simulink model "DiagramaDeSimulacao"  (R2019a)
settings: Solver=VariableStepAuto  StartTime=0.0  StopTime=210  RelTol=1e-3
values from neighbouring files (symbols this model uses):
  k1 = 6.01    [scriptDeSimulacao.m]
  k2 = 0.8433    [scriptDeSimulacao.m]
  k3 = 0.1123    [scriptDeSimulacao.m]
  V = 100    [scriptDeSimulacao.m]
libraries: powerlib_meascontrol x1
settings Model: Creator=Usuario  LastModifiedBy=Usuario

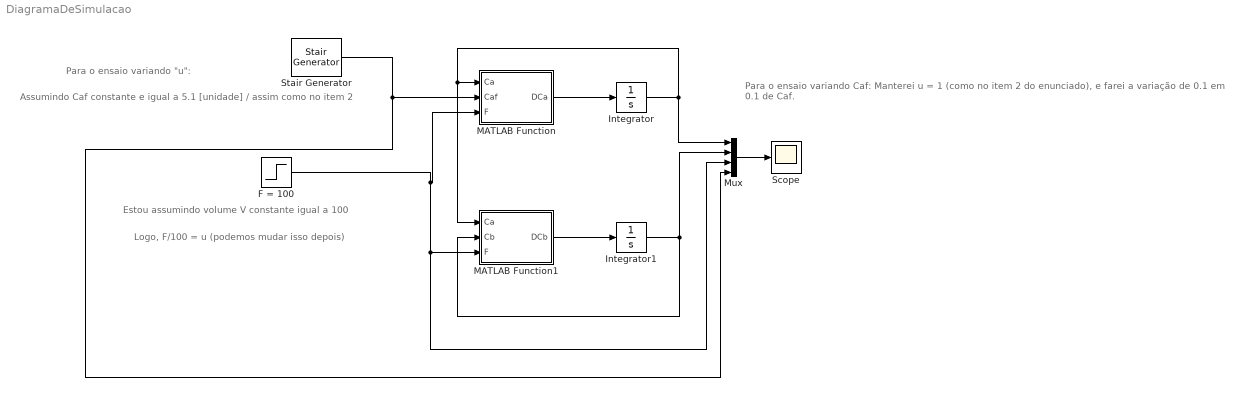
== system DiagramaDeSimulacao ==
  note: Para o ensaio variando Caf: Manterei u = 1 (como no item 2 do enunciado), e farei a variação de 0.1 em 0.1 de Caf.
  note: Para o ensaio variando "u":
  note: Assumindo Caf constante e igual a 5.1 [unidade] / assim como no item 2
  note: Logo, F/100 = u (podemos mudar isso depois)
  note: Estou assumindo volume V constante igual a 100
  F = 100 : Step  Time=0  After=100  SampleTime=0
  Integrator : Integrator
  Integrator1 : Integrator
  MATLAB Function : MATLAB Function  TreatAsAtomicUnit=on
  MATLAB Function1 : MATLAB Function  TreatAsAtomicUnit=on
  Mux : Mux
  Scope : Scope
  Stair Generator : powerlib_meascontrol/Pulse & Signal Generators/Stair Generator  t=[0, 10, 20, 30, 40, 50, 60, 70, 80, 90, 100, 110, 120, 130, 140, 150, 160, 170, 180, 190, 200]  e=[4, 4.1, 4.2, 4.3, 4.4, 4.5, 4.6, 4.7, 4.8, 4.9, 5, 5.1, 5.2, 5.3, 5.4, 5.5, 5.6, 5.7, 5.8, 5.9, 6]  Ts=0.1
      settings: SourceProductName=Simscape Electrical
  wires:
  MATLAB Function/1(DCa) -> Integrator/1
  MATLAB Function1/1(DCb) -> Integrator1/1
  Integrator/1 -> Mux/1, MATLAB Function1/1(Ca), MATLAB Function/1(Ca)
  Integrator1/1 -> MATLAB Function1/2(Cb), Mux/2
  Mux/1 -> Scope/1
  F = 100/1 -> MATLAB Function1/3(F), Mux/3, MATLAB Function/3(F)
  Stair Generator/1 -> Mux/4, MATLAB Function/2(Caf)

== matlab function DiagramaDeSimulacao/MATLAB Function1 ==
  data: DCb output; Ca input; Cb input; F input; V parameter; k2 parameter; k1 parameter
function DCb = fcn(Ca,Cb,F,V, k2, k1)

DCb = k1*Ca - k2*Cb - Cb*F/V;

== matlab function DiagramaDeSimulacao/MATLAB Function ==
  data: DCa output; Ca input; Caf input; F input; k1 parameter; k3 parameter; V parameter
function DCa = fcn(Ca,Caf,F,k1, k3, V)

DCa = -k1*Ca - k3*Ca^2 + (Caf -Ca)*F/V;
